simulink model "bh_3floor_tower_STATIONARY_GROUND_impact_test"  (R2026b)
settings: Solver=daessc  StopTime=60  FixedStep=1e-4  MaxStep=0.01  RelTol=1e-4  AbsTol=1e-4  EnableMultiTasking=on
undefined symbols (not defined in the file or in its folder): F_applied, FLOOR_1_COM, FLOOR_2_COM, FLOOR_3_COM, FLOOR_G_COM, X, Y, Z
libraries: sm_lib x14, nesl_utility x8
settings Model: Creator=bhorton  LastModifiedBy=bhorton
settings SolverCC: ZeroCrossAlgorithm=Adaptive
settings DataIOCC: LimitDataPoints=on  MaxDataPoints=10000
settings OptimizationCC: LifeSpan=inf  ReuseModelBlockBuffer=off
settings DebuggingCC: AllowSymbolicDim=off  ArithmeticOperatorsInVariantConditions=warning  SFExecutionAtInitializationDiag=none  SFNoUnconditionalDefaultTransitionDiag=warning  SFUnexpectedBacktrackingDiag=warning  SubsystemReferenceDiagnosticForUnitTest=warning
settings SFSimCC: CustomCodeUndefinedFunction=UseInterfaceOnly  SimUseLocalCustomCode=off
settings RTWCC: DLArmComputeVersion=19.05  RTWUseLocalCustomCode=off
settings CodeAppCC: StateflowObjectComments=on
settings GRTTargetCC: TargetLangStandard=C89/C90 (ANSI)
settings ConfigComp: CovExternalEMLEnable=off  CovSFcnEnable=off  CovSaveCumulativeToWorkspaceVar=on  CovSaveSingleToWorkspaceVar=on
settings SimscapeCC: SimscapeLogSimulationStatistics=on  SimscapeLogType=all  SimscapeUseEnergyAccounting=off
settings ExplorerConfigSet: InternalSimMechanicsExplorerSettings=|
  | <ExplorerConfiguration>
  | 
  |   <canonicalview>default</canonicalview>
  | 
  |   <TilePanel>
  |     <TileInfo>
  |       <Tiles Columns="2" Count="3" Height="824" Rows="2" Width="1465">
  |         <Row Weight="0.500608"/>
  |         <Row Weight="0.499392"/>
  |         <Column Weight="0.5"/>
  |         <Column Weight="0.5"/>
  |         <Tile Height="2" Width="1" X="0" Y="0"/>
  |         <Tile Height="1" Width="1" X="1" Y="0"/>
  |         <Tile Height="1" Width="1" X="1" Y="1"/>
  |       </Tiles>
  |     </TileInfo>
  |     <SceneInfo>
  |       <SceneViewer>
  |         <IsThisViewStd>
  |           <IsStandardView>off</IsStandardView>
  |           <StandardViewName>Front</StandardViewName>
  |         </IsThisViewStd>
  |         <BGColor>
  |           <R>1</R>
  |           <G>1</G>
  |           <B>1</B>
  |           <A>1</A>
  |         </BGColor>
  |         <Camera>
  |           <DoPerspective>off</DoPerspective>
  |           <Position>
  |             <X>2.4310010808664955</X>
  |             <Y>-2.0038748364052568</Y>
  |             <Z>2.2814640827283044</Z>
  |           </Position>
  |           <Center>
  |             <X>0.45054108086649569</X>
  |             <Y>-0.023414836405256885</Y>
  |             <Z>0.30100408272830426</Z>
  |           </Center>
  |           <Up>
  |             <X>-0.40824829046386307</X>
  |             <Y>0.40824829046386307</Y>
  |             <Z>0.81649658092772603</Z>
  |           </Up>
  |           <XLim>0.4972078478603138</XLim>
  |           <YLim>0.4972078478603138</YLim>
  |           <ViewLimDist>0.01</ViewLimDist>
  |         </Camera>
  |       </SceneViewer>
  |       <SceneViewer>
  |         <IsThisViewStd>
  |           <IsStandardView>off</IsStandardView>
  |           <StandardViewName>Front</StandardViewName>
  |         </IsThisViewStd>
  |         <BGColor>
  |           <R>1</R>
  |           <G>1</G>
  |           <B>1</B>
  |           <A>1</A>
  |         </BGColor>
  |         <Camera>
  |           <DoPerspective>off</DoPerspective>
  |           <Position>
  |             <X>-2.8124799999999999</X>
  |             <Y>0.03083</Y>
  |             <Z>0.28292</Z>
  |           </Position>
  |           <Center>
  |             <X>0.30779000000000001</X>
  |             <Y>0.03083</Y>
  |             <Z>0.28292</Z>
  |           </Center>
  |           <Up>
  |             <X>0</X>
  |             <Y>0</Y>
  |             <Z>1</Z>
  |           </Up>
  |           <XLim>0.41671456822244696</XLim>
  |           <YLim>0.41671456822244696</YLim>
  |           <ViewLimDist>0.01</ViewLimDist>
  |         </Camera>
  |       </SceneViewer>
  |       <SceneViewer>
  |         <IsThisViewStd>
  |           <IsStandardView>off</IsStandardView>
  |           <StandardViewName>Front</StandardViewName>
  |         </IsThisViewStd>
  |         <BGColor>
  |           <R>1</R>
  |           <G>1</G>
  |           <B>1</B>
  |           <A>1</A>
  |         </BGColor>
  |         <Camera>
  |           <DoPerspective>off</DoPerspective>
  |           <Position>
  |             <X>0.39722000000000002</X>
  |             <Y>-3.0881799999999999</Y>
  |             <Z>0.32785999999999998</Z>
  |           </Position>
  |           <Center>
  |             <X>0.39722000000000002</X>
  |             <Y>0.030679999999999999</Y>
  |             <Z>0.32785999999999998</Z>
  |           </Center>
  |           <Up>
  |             <X>0</X>
  |             <Y>0</Y>
  |             <Z>1</Z>
  |           </Up>
  |           <XLim>0.38570601860733911</XLim>
  |           <YLim>0.38570601860733911</YLim>
  |           <ViewLimDist>0.01</ViewLimDist>
  |         </Camera>
  |       </SceneViewer>
  |     </SceneInfo>
  |   </TilePanel>
  | 
  |   <MechEditorPanel>
  |     <GfxPanelCameraMap/>
  |     <Cameras/>
  |     <VideoCreator>
  |       <IncludeTiles>All</IncludeTiles>
  |       <IncludeTime>on</IncludeTime>
  |       <IncludeWorldFrame>off</IncludeWorldFrame>
  |       <PlaybackSpeedRatio>1</PlaybackSpeedRatio>
  |       <FrameRate>30</FrameRate>
  |       <FrameSize>auto</FrameSize>
  |       <VideoFormat>UncompressedAVI</VideoFormat>
  |     </VideoCreator>
  |   </MechEditorPanel>
  | 
  |   <PlaybackSettings>
  |     <PlaybackSpeedFactor>1</PlaybackSpeedFactor>
  |   </PlaybackSettings>
  | 
  | </ExplorerConfiguration>

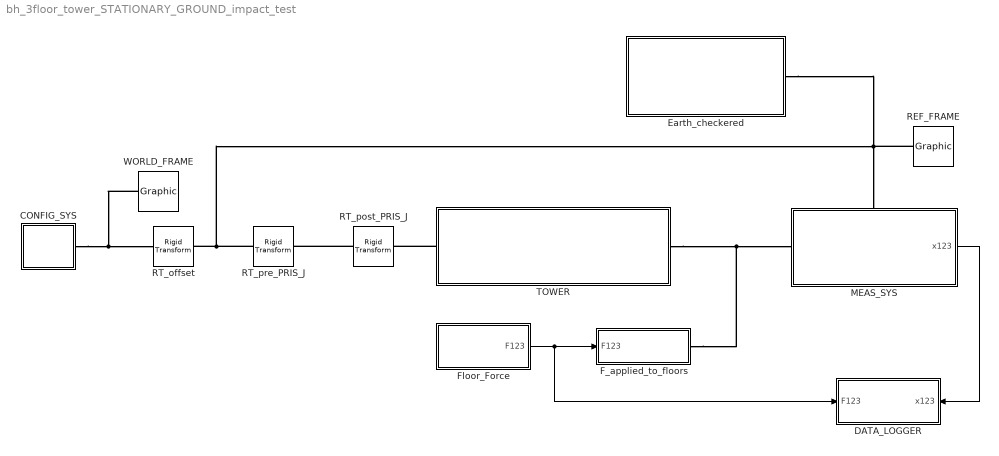
== system bh_3floor_tower_STATIONARY_GROUND_impact_test ==
  CONFIG_SYS : Subsystem
  DATA_LOGGER : Subsystem
      settings: PortSchema="{\"entries\":[{\"content\":{\"sides\":[{\"content\":{\"connectorIds\":[\"In1\"]},\"type\":\"ConnectorPlacement.EquallySpacedRectSide\",\"uuid\":\"3a1e0e0a-91b7-4f2c-a7bf-a7bd9043f7b6\"},{\"content\":{\"connectorIds\":[\"In2\"],\"side\":\"RIGHT\"},\"type\":\"ConnectorPlacement.EquallySpacedRectSide\",\"uuid\":\"78cae997-15a9-4a16-bec8-c581ca86035d\"},{\"content\":{\"side\":\"TOP\"},\"type\":\"ConnectorPlacement.EquallySpacedRectSide\",\"uuid\":\"2572a9ba-3ea9-491a-8470-66d70f2d343e\"}]},\"type\":\"ConnectorPlacement.EquallySpacedConnector\",\"uuid\":\"47241008-7b30-43ad-93f7-b59de2b7181b\"}],\"packageUris\":[\"http://schema.mathworks.com/mf0/Connector/R2020b\"],\"version\":\"1.0\"}"
  Earth_checkered : Subsystem  ReferencedSubsystem=COMP_SYS_earth_checkered
  F_applied_to_floors : Subsystem
  Floor_Force : Subsystem
  MEAS_SYS : Subsystem
      settings: PortSchema="{\"entries\":[{\"content\":{\"sides\":[{\"content\":{\"connectorIds\":[\"LConn1\"]},\"type\":\"ConnectorPlacement.EquallySpacedRectSide\",\"uuid\":\"21e9ad2b-bb8e-44e6-80e2-6778ff4dd635\"},{\"content\":{\"connectorIds\":[\"Out1\"],\"side\":\"RIGHT\"},\"type\":\"ConnectorPlacement.EquallySpacedRectSide\",\"uuid\":\"947f54f3-3be3-4ef4-b1bc-75d5ad0851bc\"},{\"content\":{\"connectorIds\":[\"LConn2\"],\"side\":\"TOP\"},\"type\":\"ConnectorPlacement.EquallySpacedRectSide\",\"uuid\":\"4e501d42-024f-4ef4-9f52-d57e50c3edc7\"}]},\"type\":\"ConnectorPlacement.EquallySpacedConnector\",\"uuid\":\"9e1969c4-c0b0-4b53-8df4-c26c3fb6ae00\"}],\"packageUris\":[\"http://schema.mathworks.com/mf0/Connector/R2020b\"],\"version\":\"1.0\"}"
  REF_FRAME : sm_lib/Body Elements/Graphic  GraphicType=Marker  MarkerShape=Frame  MarkerSize=25  GraphicVisPropType=SimpleVisualProperties  GraphicDiffuseColor=[0.3333 1 0.498]  GraphicOpacity=1  GraphicSpecularColor=[0.5 0.5 0.5 1.0]  GraphicAmbientColor=[0.15 0.15 0.15 1.0]  GraphicEmissiveColor=[0.0 0.0 0.0 1.0]  GraphicShininess=75
  RT_offset : sm_lib/Frames and Transforms/Rigid Transform  RotationMethod=None  FollAlignAxisA=+X  BaseAlignAxisA=+Y  FollAlignAxisB=+Y  BaseAlignAxisB=+Z  RotationStandardAxis=+Z  RotationAngle=0  RotationAngleUnits=deg  RotationArbitraryAxis=[0 0 1]  RotationSequenceAxes=FollowerAxes  RotationSequence=XYX  RotationSequenceAngles=[0 0 0]  RotationSequenceAnglesUnits=deg  RotationMatrix=[1 0 0;0 1 0;0 0 1]  Quaternion=[1 0 0 0]  TranslationMethod=StandardAxis  TranslationCartesianOffset=[0 0 0]  TranslationCartesianOffsetUnits=m  TranslationStandardAxis=+X  TranslationStandardOffset=0.5  TranslationStandardOffsetUnits=m  TranslationROffset=0  TranslationROffsetUnits=m  TranslationThetaOffset=0  TranslationThetaOffsetUnits=deg  TranslationZOffset=0  TranslationZOffsetUnits=m
  RT_post_PRIS_J : sm_lib/Frames and Transforms/Rigid Transform  RotationMethod=AlignedAxes  FollAlignAxisA=+Y  BaseAlignAxisA=+Y  FollAlignAxisB=+X  BaseAlignAxisB=+Z  RotationStandardAxis=+Z  RotationAngle=0  RotationAngleUnits=deg  RotationArbitraryAxis=[0 0 1]  RotationSequenceAxes=FollowerAxes  RotationSequence=XYX  RotationSequenceAngles=[0 0 0]  RotationSequenceAnglesUnits=deg  RotationMatrix=[1 0 0;0 1 0;0 0 1]  Quaternion=[1 0 0 0]  TranslationMethod=None  TranslationCartesianOffset=[0 0 0]  TranslationCartesianOffsetUnits=m  TranslationStandardAxis=+Z  TranslationStandardOffset=0  TranslationStandardOffsetUnits=m  TranslationROffset=0  TranslationROffsetUnits=m  TranslationThetaOffset=0  TranslationThetaOffsetUnits=deg  TranslationZOffset=0  TranslationZOffsetUnits=m
  RT_pre_PRIS_J : sm_lib/Frames and Transforms/Rigid Transform  RotationMethod=AlignedAxes  FollAlignAxisA=+Y  BaseAlignAxisA=+Y  FollAlignAxisB=+Z  BaseAlignAxisB=+X  RotationStandardAxis=+Z  RotationAngle=0  RotationAngleUnits=deg  RotationArbitraryAxis=[0 0 1]  RotationSequenceAxes=FollowerAxes  RotationSequence=XYX  RotationSequenceAngles=[0 0 0]  RotationSequenceAnglesUnits=deg  RotationMatrix=[1 0 0;0 1 0;0 0 1]  Quaternion=[1 0 0 0]  TranslationMethod=None  TranslationCartesianOffset=[0 0 0]  TranslationCartesianOffsetUnits=m  TranslationStandardAxis=+Z  TranslationStandardOffset=0  TranslationStandardOffsetUnits=m  TranslationROffset=0  TranslationROffsetUnits=m  TranslationThetaOffset=0  TranslationThetaOffsetUnits=deg  TranslationZOffset=0  TranslationZOffsetUnits=m
  TOWER : Subsystem  ReferencedSubsystem=COMP_3floor_flex_TOWER
  WORLD_FRAME : sm_lib/Body Elements/Graphic  GraphicType=Marker  MarkerShape=Frame  MarkerSize=25  GraphicVisPropType=SimpleVisualProperties  GraphicDiffuseColor=[0 0 0]  GraphicOpacity=1  GraphicSpecularColor=[0.5 0.5 0.5 1.0]  GraphicAmbientColor=[0.15 0.15 0.15 1.0]  GraphicEmissiveColor=[0.0 0.0 0.0 1.0]  GraphicShininess=75
  wires:
  Floor_Force/1(F123) -> DATA_LOGGER/1(F123), F_applied_to_floors/1(F123)
  MEAS_SYS/1(x123) -> DATA_LOGGER/2(x123)
  connections:
  RT_pre_PRIS_J/LConn1 -- Earth_checkered/RConn1 -- REF_FRAME/RConn1 -- MEAS_SYS/LConn2 -- RT_offset/RConn1
  WORLD_FRAME/RConn1 -- CONFIG_SYS/LConn1 -- RT_offset/LConn1
  TOWER/LConn1 -- RT_post_PRIS_J/RConn1
  TOWER/RConn1 -- F_applied_to_floors/RConn1 -- MEAS_SYS/LConn1
  RT_post_PRIS_J/LConn1 -- RT_pre_PRIS_J/RConn1

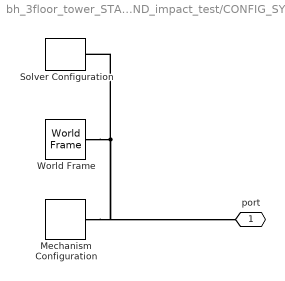
== system bh_3floor_tower_STATIONARY_GROUND_impact_test/CONFIG_SYS ==
  Mechanism Configuration : sm_lib/Utilities/Mechanism Configuration  UniformGravity=Constant  GravityVector=[0 0 -9.80665]  GravityVectorUnits=m/s^2  LinearizationDelta=0.001  JointModeTransitionNonlinearIterations=2
  Solver Configuration : nesl_utility/Solver Configuration  PhysicalDomain=network_engine_domain  SubClassName=solver  LeftPortType=input  RightPortType=generic  Tones=[]  Harmonics=[]  SimulateNoise=off  Profile=off  UseLocalSampling=off  EnableSwitchedLinearOptims=on  FrequencyDomain=off  UseCCode=off  RelTol=0.001  AbsTol=1e-06  MinStep=1e-09  ToWorkspace=off  RevertToSquareIcSolve=off  NumHomotopyIterations=100  PhasorMode=off  PhasorModeNumHarmonics=1  ConsistencySolver=NEWTON_XTOL_AFTER_FTOL  CanonicalOrdering=UNORDERED  OptimizeIntermediates=UNOPTIMIZED  MulticoreSolverChoice=BACKWARD_EULER  IndexReductionMethod=DerivativeReplacement  DoDC=off  ResidualTolerance=1e-09  ConsistencyTolSource=GLOBAL  ConsistencyAbsTol=1e-5  ConsistencyRelTol=1e-5  ConsistencyTolFactor=1e-2  UseLocalSolver=off  LocalSolverChoice=NE_BACKWARD_EULER_ADVANCER  ResolveIndetEquations=on  FunctionEvalNumThread=1  LocalSolverSampleTime=0.001  DoFixedCost=off  MaxNonlinIter=3  MaxModeIter=2  ComputeImpulses=off  ImpulseIterations=2  LinearAlgebra=Sparse  LinearAlgebraNumThread=0  EquationFormulation=NE_TIME_EF  DelaysMemoryBudget=1024  AutomaticFiltering=on  FilteringTimeConstant=0.001  PartitionStorageMethod=AS_NEEDED  PartitionMemoryBudget=1024  PartitionMethod=FAST  MultibodyUseLocalSolver=off  MultibodyLocalSolverChoice=ODE5  MultibodyLocalSolverSampleTime=0.001
  World Frame : sm_lib/Frames and Transforms/World Frame
  port : PMIOPort  Side=Left
  connections:
  World Frame/RConn1 -- Mechanism Configuration/RConn1 -- port/RConn1 -- Solver Configuration/RConn1

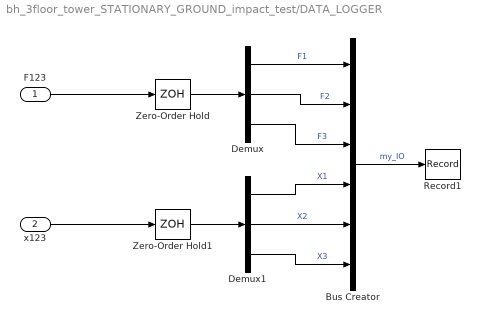
== system bh_3floor_tower_STATIONARY_GROUND_impact_test/DATA_LOGGER ==
  F123 : Inport
  x123 : Inport  Port=2
  Bus Creator : BusCreator  Inputs=6
  Demux : Demux  Outputs=3
  Demux1 : Demux  Outputs=3
  Record1 : Record  NumPorts=1.0  Filename=bh_IMPACT_TEST.xlsx  RecordToFile=on  FileSettingsInternal="{\"entries\":[{\"content\":{\"excelSettings\":{\"content\":{},\"type\":\"Streamout.ExcelSettings\"},\"parquetSettings\":{\"content\":{},\"type\":\"Streamout.ParquetSettings\"}},\"type\":\"Streamout.FileSettingStorage\",\"uuid\":\"\"}],\"packageUris\":[\"http:\\/\\/schema.mathworks.com\\/mf0\\/streamout_blocks\\/R2020a\"],\"version\":\"1.0\"}"  FrameSettings=0  SignalsInternal="{\"entries\":[{\"content\":{\"signals\":[{\"content\":{\"blockPath\":[],\"dimensions\":[1],\"domain\":\"\",\"hasChildren\":true,\"lineColor\":\"#b746ff\",\"lineWidth\":2,\"port\":1,\"signalID\":1,\"signalName\":\"my_IO\"},\"type\":\"RecordBlkView.Signal\",\"uuid\":\"\"},{\"content\":{\"blockPath\":[],\"dimensions\":[1,1],\"domain\":\"\",\"leafPath\":\"my_IO.F1\",\"lineColor\":\"#7e2f8e\",\"lineWidth\":2,\"parentID\":1,\"plots\":[ 1 ],\"port\":1,\"signalID\":2,\"signalName\":\"my_IO.F1\"},\"type\":\"RecordBlkView.Signal\",\"uuid\":\"\"},{\"content\":{\"blockPath\":[],\"dimensions\":[1,1],\"domain\":\"\",\"leafPath\":\"my_IO.F2\",\"lineColor\":\"#77ac30\",\"lineWidth\":2,\"parentID\":1,\"plots\":[ 1 ],\"port\":1,\"signalID\":3,\"signalName\":\"my_IO.F2\"},\"type\":\"RecordBlkView.Signal\",\"uuid\":\"\"},{\"content\":{\"blockPath\":[],\"dimensions\":[1,1],\"domain\":\"\",\"leafPath\":\"my_IO.F3\",\"lineColor\":\"#4dbeee\",\"lineWidth\":2,\"parentID\":1,\"plots\":[ 1 ],\"port\":1,\"signalID\":4,\"signalName\":\"my_IO.F3\"},\"type\":\"RecordBlkView.Signal\",\"uuid\":\"\"},{\"content\":{\"blockPath\":[],\"dimensions\":[1],\"domain\":\"\",\"leafPath\":\"my_IO.X1\",\"lineColor\":\"#a2142f\",\"lineWidth\":2,\"parentID\":1,\"plots\":[ 1 ],\"port\":1,\"signalID\":5,\"signalName\":\"my_IO.X1\"},\"type\":\"RecordBlkView.Signal\",\"uuid\":\"\"},{\"content\":{\"blockPath\":[],\"dimensions\":[1],\"domain\":\"\",\"leafPath\":\"my_IO.X2\",\"lineColor\":\"#139fff\",\"lineWidth\":2,\"parentID\":1,\"plots\":[ 1 ],\"port\":1,\"signalID\":6,\"signalName\":\"my_IO.X2\"},\"type\":\"RecordBlkView.Signal\",\"uuid\":\"\"},{\"content\":{\"blockPath\":[],\"dimensions\":[1],\"domain\":\"\",\"leafPath\":\"my_IO.X3\",\"lineColor\":\"#ff6929\",\"lineWidth\":2,\"parentID\":1,\"plots\":[ 1 ],\"port\":1,\"signalID\":7,\"signalName\":\"my_IO.X3\"},\"type\":\"RecordBlkView.Signal\",\"uuid\":\"\"}]},\"type\":\"RecordBlkView.InputSignals\",\"uuid\":\"\"}],\"packageUris\":[\"http:\\/\\/schema.mathworks.com\\/mf0\\/streamout_blocks\\/R2020a\"],\"version\":\"1.0\"}"  VisualizationBindings="{\"sparklinesplugin\":{\"info\":[{\"bindingParametersList\":[],\"subplotID\":1}]}}"
  Zero-Order Hold : ZeroOrderHold  SampleTime=0.01
      settings: AttributesFormatString=dT = %<SampleTime>
  Zero-Order Hold1 : ZeroOrderHold  SampleTime=0.01
      settings: AttributesFormatString=dT = %<SampleTime>
  wires:
  F123/1 -> Zero-Order Hold/1
  x123/1 -> Zero-Order Hold1/1
  Zero-Order Hold1/1 -> Demux1/1
  Zero-Order Hold/1 -> Demux/1
  Demux1/1 -> Bus Creator/4  "X1"
  Demux1/2 -> Bus Creator/5  "X2"
  Demux1/3 -> Bus Creator/6  "X3"
  Demux/1 -> Bus Creator/1  "F1"
  Demux/2 -> Bus Creator/2  "F2"
  Demux/3 -> Bus Creator/3  "F3"
  Bus Creator/1 -> Record1/1  "my_IO"

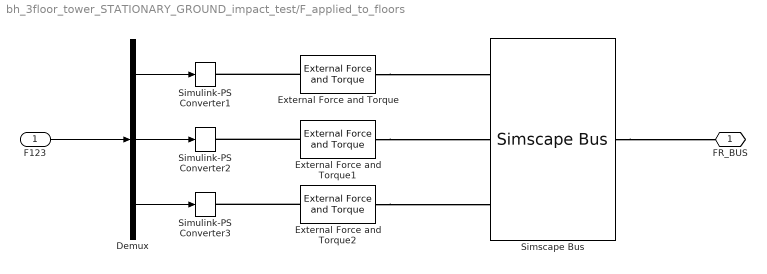
== system bh_3floor_tower_STATIONARY_GROUND_impact_test/F_applied_to_floors ==
  F123 : Inport
  Demux : Demux  Outputs=3
  External Force and Torque : sm_lib/Forces and Torques/External Force and Torque  EnableForceX=on  EnableForceY=off  EnableForceZ=off  EnableForce=off  ForceResolutionFrame=AttachedFrame  EnableTorqueX=off  EnableTorqueY=off  EnableTorqueZ=off  EnableTorque=off  TorqueResolutionFrame=AttachedFrame
  External Force and Torque1 : sm_lib/Forces and Torques/External Force and Torque  EnableForceX=on  EnableForceY=off  EnableForceZ=off  EnableForce=off  ForceResolutionFrame=AttachedFrame  EnableTorqueX=off  EnableTorqueY=off  EnableTorqueZ=off  EnableTorque=off  TorqueResolutionFrame=AttachedFrame
  External Force and Torque2 : sm_lib/Forces and Torques/External Force and Torque  EnableForceX=on  EnableForceY=off  EnableForceZ=off  EnableForce=off  ForceResolutionFrame=AttachedFrame  EnableTorqueX=off  EnableTorqueY=off  EnableTorqueZ=off  EnableTorque=off  TorqueResolutionFrame=AttachedFrame
  Simscape Bus : SimscapeBus  HierarchyStrings=FLOOR_1_COM;FLOOR_2_COM;FLOOR_3_COM
  Simulink-PS Converter1 : nesl_utility/Simulink-PS Converter  PhysicalDomain=network_engine_domain  SubClassName=ps_input  LeftPortType=input  RightPortType=output  PseudoPeriodic=off  Frequencies=[]  NoiseDistribution=none  NoiseParameters=[]  Unit=N  AffineConversion=off  FilteringAndDerivatives=provide  SimscapeFilterOrder=2  InputFilterTimeConstant=0.001  UdotUserProvided=0
  Simulink-PS Converter2 : nesl_utility/Simulink-PS Converter  PhysicalDomain=network_engine_domain  SubClassName=ps_input  LeftPortType=input  RightPortType=output  PseudoPeriodic=off  Frequencies=[]  NoiseDistribution=none  NoiseParameters=[]  Unit=N  AffineConversion=off  FilteringAndDerivatives=provide  SimscapeFilterOrder=2  InputFilterTimeConstant=0.001  UdotUserProvided=0
  Simulink-PS Converter3 : nesl_utility/Simulink-PS Converter  PhysicalDomain=network_engine_domain  SubClassName=ps_input  LeftPortType=input  RightPortType=output  PseudoPeriodic=off  Frequencies=[]  NoiseDistribution=none  NoiseParameters=[]  Unit=N  AffineConversion=off  FilteringAndDerivatives=provide  SimscapeFilterOrder=2  InputFilterTimeConstant=0.001  UdotUserProvided=0
  FR_BUS : PMIOPort  Side=Right
  wires:
  Demux/1 -> Simulink-PS Converter1/1
  F123/1 -> Demux/1
  Demux/3 -> Simulink-PS Converter3/1
  Demux/2 -> Simulink-PS Converter2/1
  connections:
  Simscape Bus/RConn1 -- FR_BUS/RConn1
  External Force and Torque/RConn1 -- Simscape Bus/LConn1
  External Force and Torque/LConn1 -- Simulink-PS Converter1/RConn1
  External Force and Torque1/LConn1 -- Simulink-PS Converter2/RConn1
  External Force and Torque2/LConn1 -- Simulink-PS Converter3/RConn1
  External Force and Torque1/RConn1 -- Simscape Bus/LConn2
  External Force and Torque2/RConn1 -- Simscape Bus/LConn3

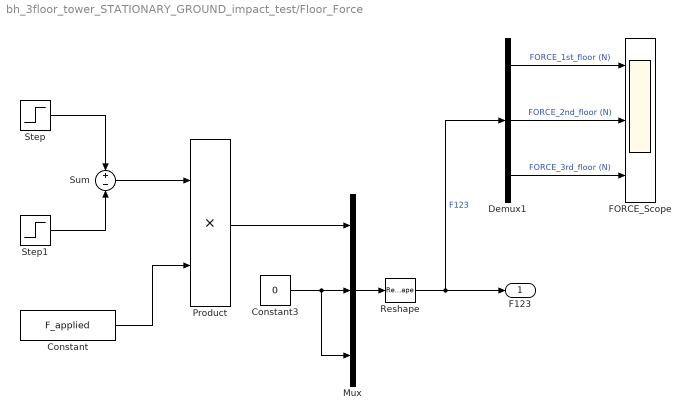
== system bh_3floor_tower_STATIONARY_GROUND_impact_test/Floor_Force ==
  Constant : Constant  Value=F_applied
  Constant3 : Constant  Value=0
  Demux1 : Demux  Outputs=3
  FORCE_Scope : Scope  NumInputPorts=3
      settings: ActiveDisplayYMinimum=-0.026703081424579757  ActiveDisplayYMaximum=0.027552885742231394
  Mux : Mux  Inputs=3
  Product : Product
  Reshape : Reshape  OutputDimensionality=Column vector (2-D)
  Step : Step  SampleTime=0
      settings: AttributesFormatString=T_step =%<Time>
  Step1 : Step  Time=1+0.01  SampleTime=0
      settings: AttributesFormatString=T_step =%<Time>
  Sum : Sum  Inputs=+|-
  F123 : Outport
  wires:
  Mux/1 -> Reshape/1
  Step/1 -> Sum/1
  Step1/1 -> Sum/2
  Sum/1 -> Product/1
  Constant/1 -> Product/2
  Product/1 -> Mux/1
  Constant3/1 -> Mux/3, Mux/2
  Demux1/2 -> FORCE_Scope/2  "FORCE_2nd_floor (N)"
  Demux1/1 -> FORCE_Scope/1  "FORCE_1st_floor (N)"
  Demux1/3 -> FORCE_Scope/3  "FORCE_3rd_floor (N)"
  Reshape/1 -> Demux1/1, F123/1  "F123"

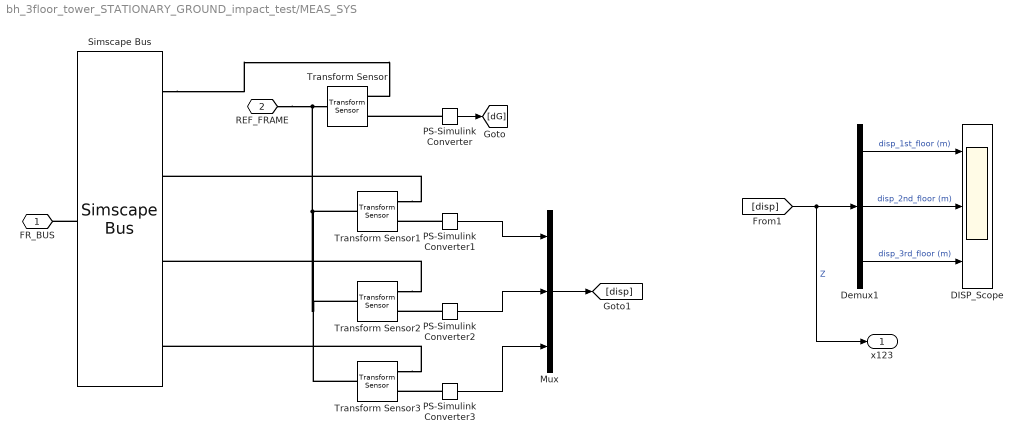
== system bh_3floor_tower_STATIONARY_GROUND_impact_test/MEAS_SYS ==
  DISP_Scope : Scope  NumInputPorts=3
      settings: ActiveDisplayYMinimum=-0.026703081424579757  ActiveDisplayYMaximum=0.027552885742231394
  Demux1 : Demux  Outputs=3
  Mux : Mux  Inputs=3
  PS-Simulink Converter{,1..3} (4 alike) : nesl_utility/PS-Simulink Converter  PhysicalDomain=network_engine_domain  SubClassName=ps_output  LeftPortType=input  RightPortType=output  PseudoPeriodic=off  Frequencies=[]  VectorFormat=inherit  Unit=m  AffineConversion=off
  Simscape Bus : SimscapeBus  HierarchyStrings=FLOOR_G_COM;FLOOR_1_COM;FLOOR_2_COM;FLOOR_3_COM
  Transform Sensor{,1..3} (4 alike) : sm_lib/Frames and Transforms/Transform Sensor  ObservationFrame=World  ExpressedInFrame=World  RotationSequence=XYX  SenseAngle=off  SenseAxis=off  SenseQ=off  SenseR=off  SenseRotationSequence=off  SenseOmegaX=off  SenseOmegaY=off  SenseOmegaZ=off  SenseOmega=off  SenseQDot=off  SenseRDot=off  SenseRotationSequenceDot=off  SenseAlphaX=off  SenseAlphaY=off  SenseAlphaZ=off  SenseAlpha=off  SenseQDDot=off  SenseRDDot=off  SenseX=on  SenseY=off  SenseZ=off  SenseXYZ=off  SenseRad=off  SenseAzim=off  SenseDist=off  SenseInc=off  SenseXDot=off  SenseYDot=off  SenseZDot=off  SenseXYZDot=off  SenseRadDot=off  SenseAzimDot=off  SenseDistDot=off  SenseIncDot=off  SenseXDDot=off  SenseYDDot=off  SenseZDDot=off  SenseXYZDDot=off  SenseRadDDot=off  SenseAzimDDot=off  SenseDistDDot=off  SenseIncDDot=off
  FR_BUS : PMIOPort  Side=Left
  REF_FRAME : PMIOPort  Port=2  Side=Left
  x123 : Outport
  wires:
  PS-Simulink Converter/1 -> [dG]
  Demux1/3 -> DISP_Scope/3  "disp_3rd_floor (m)"
  Demux1/1 -> DISP_Scope/1  "disp_1st_floor (m)"
  [disp] -> x123/1, Demux1/1  "Z"
  Demux1/2 -> DISP_Scope/2  "disp_2nd_floor (m)"
  PS-Simulink Converter1/1 -> Mux/1
  PS-Simulink Converter2/1 -> Mux/2
  PS-Simulink Converter3/1 -> Mux/3
  Mux/1 -> [disp]
  connections:
  REF_FRAME/RConn1 -- Transform Sensor3/LConn1 -- Transform Sensor2/LConn1 -- Transform Sensor1/LConn1 -- Transform Sensor/LConn1
  Simscape Bus/RConn1 -- FR_BUS/RConn1
  Simscape Bus/LConn1 -- Transform Sensor/RConn1
  PS-Simulink Converter/LConn1 -- Transform Sensor/RConn2
  PS-Simulink Converter1/LConn1 -- Transform Sensor1/RConn2
  Transform Sensor1/RConn1 -- Simscape Bus/LConn2
  Transform Sensor2/RConn1 -- Simscape Bus/LConn3
  PS-Simulink Converter2/LConn1 -- Transform Sensor2/RConn2
  PS-Simulink Converter3/LConn1 -- Transform Sensor3/RConn2
  Transform Sensor3/RConn1 -- Simscape Bus/LConn4
